simulink model "Subsystem0"  (R2020a)
settings: Solver=VariableStepAuto  StartTime=0.0  StopTime=10.0  RelTol=1e-3
model workspace (MAT data in the model file):
  A = 2
  B = 2
settings Model: DataDictionary=new_data.sldd  Creator=Riyansh  LastModifiedBy=Riyansh
settings DataIOCC: SaveOutput=off  SaveTime=off

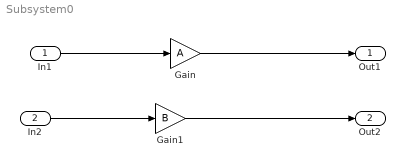
== system Subsystem0 ==
  In1 : Inport  OutDataTypeStr=double  PortDimensions=1
  In2 : Inport  Port=2  OutDataTypeStr=double  PortDimensions=1
  Gain : Gain  Gain=A
  Gain1 : Gain  Gain=B
  Out1 : Outport  OutDataTypeStr=double  PortDimensions=1
  Out2 : Outport  Port=2  OutDataTypeStr=double  PortDimensions=1
  wires:
  Gain/1 -> Out1/1
  In1/1 -> Gain/1
  In2/1 -> Gain1/1
  Gain1/1 -> Out2/1
